simulink model "c1_chirp_filter"  (R2020b)
settings: Solver=FixedStepDiscrete  StartTime=0.0  StopTime=stopTime  FixedStep=2.0833333333333333e-05  RelTol=1e-3
values from neighbouring files (symbols this model uses):
  C1initphase = C1initphase + atan(CF/(-rzero))-atan((CF-pimag(2*i-1))/(-preal(2*i-1)))-atan((CF+pimag(2*i-1))/(-preal(2*i-1)))    [c1_chirp_parameter.m]
  CF = 2*pi*cf    [c1_chirp_parameter.m]
  cihc = 1    [modelparameters.m]
  fs_bilinear = 2*pi*cf/tan(2*pi*cf*tdres/2)    [c1_chirp_parameter.m]
  norm_gainc1 = (sqrt(C1gain_norm))/((sqrt(CF^2+rzero^2))^order_of_zero)    [c1_chirp_parameter.m]
  order_of_zero = half_order_pole    (= 5)    [c1_chirp_parameter.m]
  pimag = zeros(11,1)    [c1_chirp_parameter.m]
  preal = zeros(11,1)    [c1_chirp_parameter.m]
settings Model: Creator=Ross  LastModifiedBy=wickh
settings DataIOCC: SaveOutput=off  SaveTime=off  ReturnWorkspaceOutputs=off
settings OptimizationCC: BlockReduction=off  ConditionallyExecuteInputs=off  DefaultParameterBehavior=Inlined
settings DebuggingCC: ReadBeforeWriteMsg=DisableAll  WriteAfterWriteMsg=DisableAll  WriteAfterReadMsg=DisableAll  AlgebraicLoopMsg=error  MultiTaskDSMMsg=none  SingleTaskRateTransMsg=error  PregeneratedLibrarySubsystemCodeDiagnostic=none  ArithmeticOperatorsInVariantConditions=warning
settings HardwareCC: ProdBitPerPointer=32  ProdBitPerSizeT=32  ProdBitPerPtrDiffT=32  ProdLargestAtomicFloat=None  ProdIntDivRoundTo=Undefined  ProdEndianess=Unspecified  ProdWordSize=32  ProdHWDeviceType=ASIC/FPGA->ASIC/FPGA  TargetBitPerPointer=64  TargetBitPerSizeT=64  TargetBitPerPtrDiffT=64  TargetLongLongMode=on  TargetIntDivRoundTo=Zero  TargetEndianess=LittleEndian  TargetWordSize=64  TargetHWDeviceType=Custom Processor->MATLAB Host Computer  ProdEqTarget=off
settings ModelReferenceCC: UpdateModelReferenceTargets=IfOutOfDate  ModelReferenceNumInstancesAllowed=Single
settings SFSimCC: SFSimEcho=off  SimUseLocalCustomCode=off  CustomCodeUndefinedFunction=UseInterfaceOnly
settings RTWCC: RTWUseLocalCustomCode=off

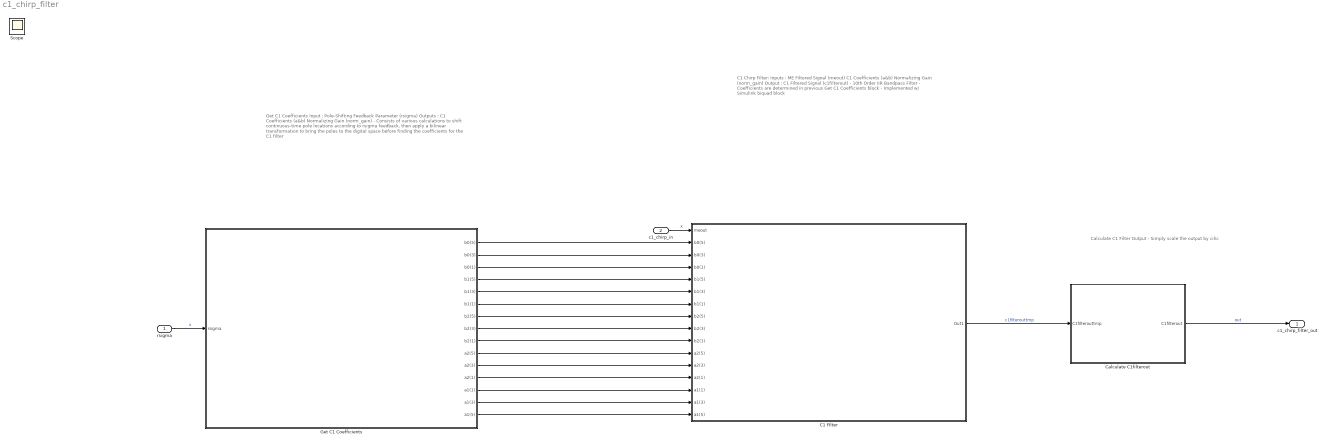
== system c1_chirp_filter ==
  note: Calculate C1 Filter Output
      |
      | - Simply scale the output by cihc
  note: Get C1 Coefficients
      |
      | Input : Pole-Shifting Feedback Parameter (rsigma)
      |
      | Outputs : C1 Coefficients (a&b)
      | Normalizing Gain (norm_gain)
      |
      | - Consists of various calculations to shift continuous-time pole locations according to rsigma feedback, then apply a bilinear transformation to bring the poles to the digital space before finding the coefficients for the C1 filter
  note: C1 Chirp Filter:
      |
      | Inputs : ME Filtered Signal (meout)
      | C1 Coefficients (a&b)
      | Normalizing Gain (norm_gain)
      |
      | Output : C1 Filtered Signal (c1filterout)
      |
      | - 10th Order IIR Bandpass Filter
      |
      | - Coefficients are determined in previous Get C1 Coefficients block
      |
      | - Implemented w/ Simulink biquad block
  rsigma : Inport  OutDataTypeStr=single  PortDimensions=1  SampleTime=[2.0833333333333333e-05,0]
  c1_chirp_in : Inport  Port=2  OutDataTypeStr=single  PortDimensions=1  SampleTime=[2.0833333333333333e-05,0]
  C1 FIlter : Subsystem
  Calculate C1filterout : Subsystem
  Get C1 Coefficients : Subsystem
  c1_chirp_filter_out : Outport  OutDataTypeStr=single  PortDimensions=1  SampleTime=[2.0833333333333333e-05,0]  VectorParamsAs1DForOutWhenUnconnected=off
  Scope : Scope
  wires:
  Calculate C1filterout/1(C1filterout) -> c1_chirp_filter_out/1  "out"
  c1_chirp_in/1 -> C1 FIlter/1(meout)  "x"
  Get C1 Coefficients/7(b2(5)) -> C1 FIlter/8(b2(5))
  Get C1 Coefficients/11(a2(3)) -> C1 FIlter/12(a2(3))
  Get C1 Coefficients/8(b2(3)) -> C1 FIlter/9(b2(3))
  C1 FIlter/1(Out1) -> Calculate C1filterout/1(C1filterouttmp)  "c1filterouttmp"
  Get C1 Coefficients/14(a1(3)) -> C1 FIlter/15(a1(3))
  Get C1 Coefficients/9(b2(1)) -> C1 FIlter/10(b2(1))
  Get C1 Coefficients/10(a2(5)) -> C1 FIlter/11(a2(5))
  Get C1 Coefficients/15(a1(5)) -> C1 FIlter/16(a1(5))
  Get C1 Coefficients/5(b1(3)) -> C1 FIlter/6(b1(3))
  Get C1 Coefficients/3(b0(1)) -> C1 FIlter/4(b0(1))
  Get C1 Coefficients/12(a2(1)) -> C1 FIlter/13(a2(1))
  Get C1 Coefficients/6(b1(1)) -> C1 FIlter/7(b1(1))
  Get C1 Coefficients/1(b0(5)) -> C1 FIlter/2(b0(5))
  Get C1 Coefficients/13(a1(1)) -> C1 FIlter/14(a1(1))
  Get C1 Coefficients/4(b1(5)) -> C1 FIlter/5(b1(5))
  Get C1 Coefficients/2(b0(3)) -> C1 FIlter/3(b0(3))
  rsigma/1 -> Get C1 Coefficients/1(rsigma)  "x"

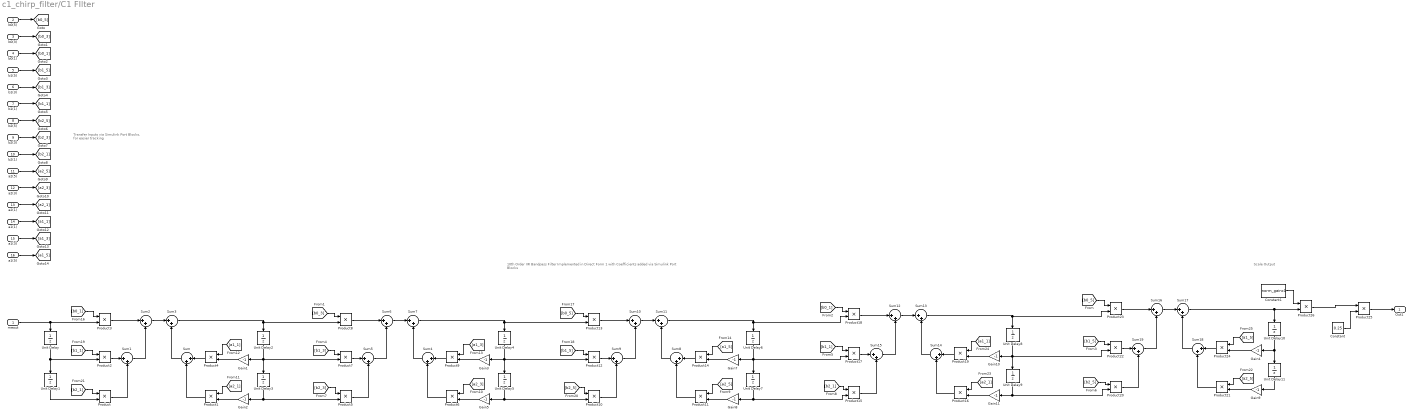
== system c1_chirp_filter/C1 FIlter ==
  note: Scale Output
  note: 10th Order IIR Bandpass Filter Implemented in Direct Form 1 with Coefficients added via Simulink Port Blocks
  note: Transfer Inputs via Simulink Port Blocks, for easier tracking
  meout : Inport
  b0(5) : Inport  Port=2
  b0(3) : Inport  Port=3
  b0(1) : Inport  Port=4
  b1(5) : Inport  Port=5
  b1(3) : Inport  Port=6
  b1(1) : Inport  Port=7
  b2(5) : Inport  Port=8
  b2(3) : Inport  Port=9
  b2(1) : Inport  Port=10
  a2(5) : Inport  Port=11
  a2(3) : Inport  Port=12
  a2(1) : Inport  Port=13
  a1(1) : Inport  Port=14
  a1(3) : Inport  Port=15
  a1(5) : Inport  Port=16
  Constant : Constant  Value=0.25  OutDataTypeStr=single  SampleTime=-1
  Constant1 : Constant  Value=norm_gainc1  OutDataTypeStr=single  SampleTime=-1
  Gain{1..5,7..11} (10 alike) : Gain  Gain=-1
  Product{,1..24} (25 alike) : Product
  Product25 : Product  OutDataTypeStr=single
  Product26 : Product  OutDataTypeStr=single
  Sum{,1..19} (20 alike) : Sum  Inputs=|++
  Unit Delay{,1,4..11} (10 alike) : UnitDelay  SampleTime=-1  HasFrameUpgradeWarning=on
  Unit Delay2 : UnitDelay  InitialCondition=1  SampleTime=-1  HasFrameUpgradeWarning=on
  Unit Delay3 : UnitDelay  InitialCondition=1  SampleTime=-1  HasFrameUpgradeWarning=on
  Out1 : Outport  VectorParamsAs1DForOutWhenUnconnected=off
  wires:
  Constant1/1 -> Product26/1
  Product26/1 -> Product25/1
  Constant/1 -> Product25/2
  Gain9/1 -> Product21/2
  Gain4/1 -> Product24/2
  Gain11/1 -> Product16/2
  Gain10/1 -> Product19/2
  Gain8/1 -> Product11/2
  Gain7/1 -> Product14/2
  Gain5/1 -> Product6/2
  Gain3/1 -> Product9/2
  Gain2/1 -> Product1/2
  Gain1/1 -> Product4/2
  a1(5)/1 -> [a1_5]
  a1(3)/1 -> [a1_3]
  a1(1)/1 -> [a1_1]
  a2(1)/1 -> [a2_1]
  a2(3)/1 -> [a2_3]
  a2(5)/1 -> [a2_5]
  b2(1)/1 -> [b2_1]
  b2(3)/1 -> [b2_3]
  b2(5)/1 -> [b2_5]
  b1(1)/1 -> [b1_1]
  b1(3)/1 -> [b1_3]
  b1(5)/1 -> [b1_5]
  b0(1)/1 -> [b0_1]
  b0(3)/1 -> [b0_3]
  b0(5)/1 -> [b0_5]
  Product1/1 -> Sum/2
  Unit Delay1/1 -> Product/2
  Sum/1 -> Sum3/2
  [a1_1] -> Product4/1
  Sum14/1 -> Sum13/2
  Unit Delay9/1 -> Gain11/1, Product20/2
  Product/1 -> Sum1/2
  [b2_1] -> Product15/1
  [b2_5] -> Product10/1
  Sum10/1 -> Sum11/1
  [a2_3] -> Product6/1
  [a2_1] -> Product16/1
  [b1_5] -> Product22/1
  Sum18/1 -> Sum17/2
  [b1_1] -> Product2/1
  Product21/1 -> Sum18/2
  Sum16/1 -> Sum17/1
  Sum9/1 -> Sum10/2
  Product6/1 -> Sum4/2
  Product13/1 -> Sum10/1
  [b1_1] -> Product17/1
  Product9/1 -> Sum4/1
  Product23/1 -> Sum16/1
  Product25/1 -> Out1/1
  Unit Delay11/1 -> Gain9/1
  [a2_5] -> Product11/1
  Unit Delay10/1 -> Gain4/1, Unit Delay11/1
  Unit Delay7/1 -> Gain8/1, Product15/2
  Product17/1 -> Sum15/1
  Unit Delay/1 -> Product2/2, Unit Delay1/1
  [a2_5] -> Product21/1
  [a1_1] -> Product19/1
  [b0_1] -> Product18/1
  [b0_5] -> Product23/1
  Sum12/1 -> Sum13/1
  [b0_3] -> Product8/1
  Sum8/1 -> Sum11/2
  Product18/1 -> Sum12/1
  Product14/1 -> Sum8/1
  [b2_5] -> Product20/1
  Sum19/1 -> Sum16/2
  Product11/1 -> Sum8/2
  Sum2/1 -> Sum3/1
  [b1_5] -> Product12/1
  Unit Delay5/1 -> Gain5/1, Product10/2
  Sum11/1 -> Unit Delay6/1, Product18/2
  Product2/1 -> Sum1/1
  meout/1 -> Unit Delay/1, Product3/2
  Product8/1 -> Sum6/1
  Product22/1 -> Sum19/1
  [a1_3] -> Product9/1
  [b0_5] -> Product13/1
  Sum6/1 -> Sum7/1
  [a1_5] -> Product24/1
  Product20/1 -> Sum19/2
  Product10/1 -> Sum9/2
  Product7/1 -> Sum5/1
  Product19/1 -> Sum14/1
  Sum4/1 -> Sum7/2
  Sum3/1 -> Unit Delay2/1, Product8/2
  Sum13/1 -> Unit Delay8/1, Product23/2
  Unit Delay4/1 -> Gain3/1, Unit Delay5/1, Product12/2
  Product5/1 -> Sum5/2
  Unit Delay3/1 -> Gain2/1, Product5/2
  Product24/1 -> Sum18/1
  [b2_1] -> Product/1
  [a2_1] -> Product1/1
  Sum7/1 -> Unit Delay4/1, Product13/2
  [b2_3] -> Product5/1
  Product3/1 -> Sum2/1
  Sum17/1 -> Unit Delay10/1, Product26/2
  Product12/1 -> Sum9/1
  Unit Delay8/1 -> Gain10/1, Unit Delay9/1, Product22/2
  Product4/1 -> Sum/1
  [b0_1] -> Product3/1
  Sum1/1 -> Sum2/2
  [b1_3] -> Product7/1
  Unit Delay6/1 -> Gain7/1, Unit Delay7/1, Product17/2
  Unit Delay2/1 -> Gain1/1, Unit Delay3/1, Product7/2
  Sum15/1 -> Sum12/2
  Sum5/1 -> Sum6/2
  Product16/1 -> Sum14/2
  Product15/1 -> Sum15/2
  [a1_5] -> Product14/1

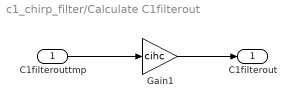
== system c1_chirp_filter/Calculate C1filterout ==
  C1filterouttmp : Inport
  Gain1 : Gain  Gain=cihc
  C1filterout : Outport  VectorParamsAs1DForOutWhenUnconnected=off
  wires:
  Gain1/1 -> C1filterout/1
  C1filterouttmp/1 -> Gain1/1

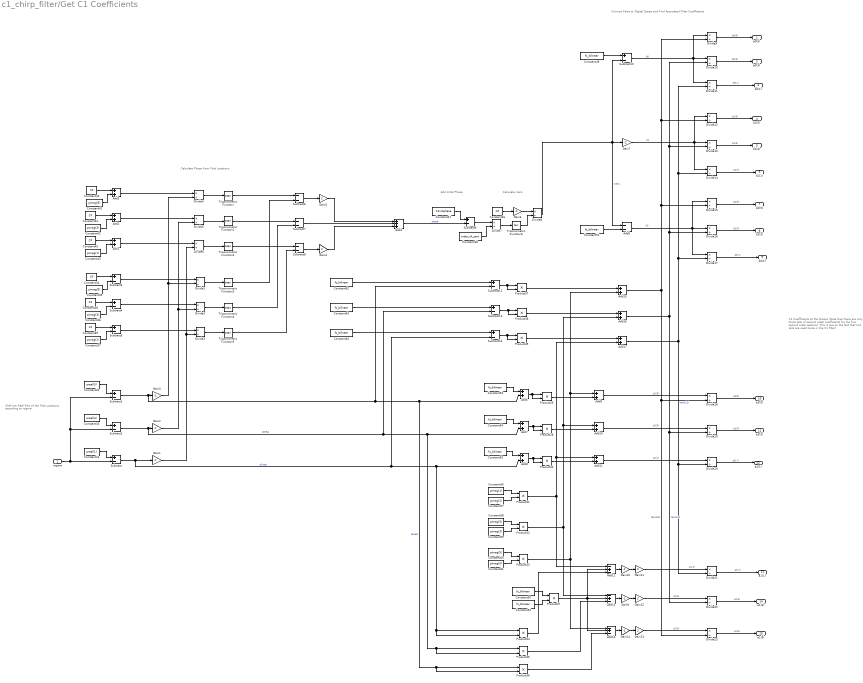
== system c1_chirp_filter/Get C1 Coefficients ==
  note: C1 Coefficients at the Output (Note that there are only three sets of second order coefficients for the five second order sections. This is due to the fact that two sets are used twice in the C1 filter)
  note: Convert Poles to Digital Spcae and Find Associated Filter Coefficients
  note: Calculate rzero
  note: Add Initial Phase
  note: Shift the Real Part of the Pole Locations according to rsigma
  note: Calculate Phase from Pole Locations
  rsigma : Inport
  Add{1..3,6..11,15..17} (12 alike) : Sum
  Add12 : Sum  Inputs=-+-
  Add13 : Sum  Inputs=-+-
  Add14 : Sum  Inputs=-+-
  Add4 : Sum  Inputs=+++
  Add5 : Sum  Inputs=--
  Constant31 : Constant  Value=preal(1)  OutDataTypeStr=single  SampleTime=-1
  Constant32 : Constant  Value=preal(5)  OutDataTypeStr=single  SampleTime=-1
  Constant33 : Constant  Value=preal(3)  OutDataTypeStr=single  SampleTime=-1
  Constant{34,38..40,44..46} (7 alike) : Constant  Value=CF  OutDataTypeStr=single  SampleTime=-1
  Constant{35,41,60..61} (4 alike) : Constant  Value=pimag(5)  OutDataTypeStr=single  SampleTime=-1
  Constant{36,42,58..59} (4 alike) : Constant  Value=pimag(3)  OutDataTypeStr=single  SampleTime=-1
  Constant{37,43,56..57} (4 alike) : Constant  Value=pimag(1)  OutDataTypeStr=single  SampleTime=-1
  Constant47 : Constant  Value=C1initphase  OutDataTypeStr=single  SampleTime=-1
  Constant48 : Constant  Value=order_of_zero  OutDataTypeStr=single  SampleTime=-1
  Constant{49..55,62..64} (10 alike) : Constant  Value=fs_bilinear  OutDataTypeStr=single  SampleTime=-1
  Divide{1..23} (23 alike) : Product  Inputs=*/  RndMeth=Zero  SaturateOnIntegerOverflow=on
  Gain{1..3,6,9..10,14} (7 alike) : Gain  Gain=-1
  Gain{4..5,11..13} (5 alike) : Gain  Gain=2
  Gain7 : Gain  Gain=-2
  Product{27..39} (13 alike) : Product
  Subtract{,1..5,9..13} (11 alike) : Sum  Inputs=+-
  Subtract6 : Sum  Inputs=--
  Subtract7 : Sum  Inputs=--
  Subtract8 : Sum  Inputs=--
  Trigonometric Function{,1..5} (6 alike) : Trigonometry  Operator=atan  ApproximationMethod=CORDIC
  Trigonometric Function6 : Trigonometry  Operator=tan  ApproximationMethod=CORDIC
  b0(5) : Outport  VectorParamsAs1DForOutWhenUnconnected=off
  b0(3) : Outport  Port=2  VectorParamsAs1DForOutWhenUnconnected=off
  b0(1) : Outport  Port=3  VectorParamsAs1DForOutWhenUnconnected=off
  b1(5) : Outport  Port=4  VectorParamsAs1DForOutWhenUnconnected=off
  b1(3) : Outport  Port=5  VectorParamsAs1DForOutWhenUnconnected=off
  b1(1) : Outport  Port=6  VectorParamsAs1DForOutWhenUnconnected=off
  b2(5) : Outport  Port=7  VectorParamsAs1DForOutWhenUnconnected=off
  b2(3) : Outport  Port=8  VectorParamsAs1DForOutWhenUnconnected=off
  b2(1) : Outport  Port=9  VectorParamsAs1DForOutWhenUnconnected=off
  a2(5) : Outport  Port=10  VectorParamsAs1DForOutWhenUnconnected=off
  a2(3) : Outport  Port=11  VectorParamsAs1DForOutWhenUnconnected=off
  a2(1) : Outport  Port=12  VectorParamsAs1DForOutWhenUnconnected=off
  a1(1) : Outport  Port=13  VectorParamsAs1DForOutWhenUnconnected=off
  a1(3) : Outport  Port=14  VectorParamsAs1DForOutWhenUnconnected=off
  a1(5) : Outport  Port=15  VectorParamsAs1DForOutWhenUnconnected=off
  wires:
  Gain14/1 -> Gain13/1
  Gain9/1 -> Gain12/1
  Gain10/1 -> Gain11/1
  Divide16/1 -> b2(3)/1  "b2(3)"
  Divide19/1 -> a2(3)/1  "a2(3)"
  Divide9/1 -> b0(5)/1  "b0(5)"
  Divide22/1 -> a1(3)/1  "a1(3)"
  Divide10/1 -> b0(3)/1  "b0(3)"
  Divide15/1 -> b2(5)/1  "b2(5)"
  Divide14/1 -> b1(1)/1  "b1(1)"
  Divide11/1 -> b0(1)/1  "b0(1)"
  Divide20/1 -> a2(1)/1  "a2(1)"
  Divide12/1 -> b1(5)/1  "b1(5)"
  Divide17/1 -> b2(1)/1  "b2(1)"
  Constant53/1 -> Add6/1
  Constant48/1 -> Divide7/2
  Constant43/1 -> Add1/2
  Constant35/1 -> Subtract3/2
  Trigonometric Function/1 -> Subtract6/1
  Constant38/1 -> Subtract4/1
  Add10/1 -> Divide19/1  "a2(3)"
  Constant64/1 -> Subtract13/1
  Constant57/1 -> Product31/2
  Constant54/1 -> Add7/1
  Constant60/1 -> Product33/1
  Constant61/1 -> Product33/2
  Constant39/1 -> Subtract5/1
  Constant36/1 -> Subtract4/2
  Divide13/1 -> b1(3)/1  "b1(3)"
  Product28/1 -> Add10/2
  Constant51/1 -> Add5/2
  Gain5/1 -> Add4/1
  Add7/1 -> Product28/1, Product28/2
  Constant56/1 -> Product31/1
  Gain4/1 -> Add4/3
  Constant45/1 -> Add1/1
  Constant34/1 -> Subtract3/1
  Subtract3/1 -> Divide1/1
  Subtract4/1 -> Divide2/1
  Add1/1 -> Divide6/1
  Subtract5/1 -> Divide3/1
  Add11/1 -> Divide20/1  "a2(1)"
  Constant50/1 -> Product27/1
  Constant37/1 -> Subtract5/2
  Add3/1 -> Divide4/1
  Subtract12/1 -> Product38/1, Product38/2
  Trigonometric Function2/1 -> Subtract8/1
  Constant49/1 -> Subtract10/1
  Constant47/1 -> Subtract9/1
  Product29/1 -> Add9/2
  Add6/1 -> Product29/1, Product29/2
  Divide7/1 -> Trigonometric Function6/1
  Divide23/1 -> a1(5)/1  "a1(5)"
  Constant55/1 -> Add8/1
  Divide1/1 -> Trigonometric Function3/1
  Divide3/1 -> Trigonometric Function5/1
  Gain3/1 -> Divide1/2, Divide4/2
  Product37/1 -> Add15/1
  Divide4/1 -> Trigonometric Function/1
  Constant42/1 -> Add2/2
  Gain13/1 -> Divide23/1  "a1(5)"
  Subtract6/1 -> Gain5/1
  Add2/1 -> Divide5/1
  Trigonometric Function1/1 -> Subtract7/1
  Gain6/1 -> Divide8/1
  Constant40/1 -> Add3/1
  Add8/1 -> Product30/1, Product30/2
  Trigonometric Function6/1 -> Divide8/2
  Constant32/1 -> Subtract1/1
  Gain12/1 -> Divide22/1  "a1(3)"
  Gain11/1 -> Divide21/1  "a1(1)"
  Subtract11/1 -> Product37/1, Product37/2
  Trigonometric Function5/1 -> Subtract8/2
  Trigonometric Function4/1 -> Subtract7/2
  Product34/1 -> Add12/3
  Divide8/1 -> Gain7/1, Add5/1, Subtract10/2  "rzero"
  Constant63/1 -> Subtract12/1
  Add16/1 -> Divide16/2, Divide13/2, Divide10/2, Divide19/2, Divide22/2  "temp(3)"
  Product35/1 -> Add13/3
  Gain7/1 -> Divide12/1, Divide13/1, Divide14/1  "b1"
  Constant44/1 -> Add2/1
  Constant41/1 -> Add3/2
  Product33/1 -> Add14/1, Add15/2, Add9/1
  Add9/1 -> Divide18/1  "a2(5)"
  Product36/1 -> Add14/3
  Trigonometric Function3/1 -> Subtract6/2
  Constant31/1 -> Subtract/1
  Subtract10/1 -> Divide9/1, Divide10/1, Divide11/1  "b0"
  Divide2/1 -> Trigonometric Function4/1
  Constant58/1 -> Product32/1
  Constant62/1 -> Subtract11/1
  Subtract7/1 -> Add4/2
  Product32/1 -> Add13/1, Add10/1, Add16/2
  Divide21/1 -> a1(1)/1  "a1(1)"
  Product39/1 -> Add17/1
  Product38/1 -> Add16/1
  Subtract13/1 -> Product39/1, Product39/2
  Product30/1 -> Add11/2
  Add4/1 -> Subtract9/2  "phase"
  Constant59/1 -> Product32/2
  Divide5/1 -> Trigonometric Function1/1
  Subtract/1 -> Gain1/1, Add8/2, Product34/2, Product34/1, Subtract13/2  "p1real"
  Subtract1/1 -> Gain3/1, Add6/2, Product36/1, Product36/2, Subtract11/2  "p5real"
  Subtract2/1 -> Gain2/1, Add7/2, Product35/1, Product35/2, Subtract12/2  "p3real"
  Product27/1 -> Add12/2, Add13/2, Add14/2
  Add14/1 -> Gain14/1
  Add15/1 -> Divide15/2, Divide12/2, Divide9/2, Divide18/2, Divide23/2  "temp(5)"
  Add13/1 -> Gain9/1
  Constant52/1 -> Product27/2
  Add12/1 -> Gain10/1
  Gain1/1 -> Divide3/2, Divide6/2
  rsigma/1 -> Subtract2/2, Subtract1/2, Subtract/2
  Subtract8/1 -> Gain4/1
  Gain2/1 -> Divide2/2, Divide5/2
  Product31/1 -> Add11/1, Add17/2, Add12/1
  Add17/1 -> Divide14/2, Divide11/2, Divide17/2, Divide20/2, Divide21/2  "temp(1)"
  Constant33/1 -> Subtract2/1
  Subtract9/1 -> Divide7/1
  Divide18/1 -> a2(5)/1  "a2(5)"
  Divide6/1 -> Trigonometric Function2/1
  Constant46/1 -> Gain6/1
  Add5/1 -> Divide15/1, Divide16/1, Divide17/1  "b2"
